simulink model "test"  (R2019a)
settings: Solver=VariableStepAuto  StartTime=0.0  StopTime=10.0  RelTol=1e-3
libraries: powerlib x9, re_lib x1, powerlib_meascontrol x1, ee_lib x1
settings Model: Creator=engma  LastModifiedBy=engma

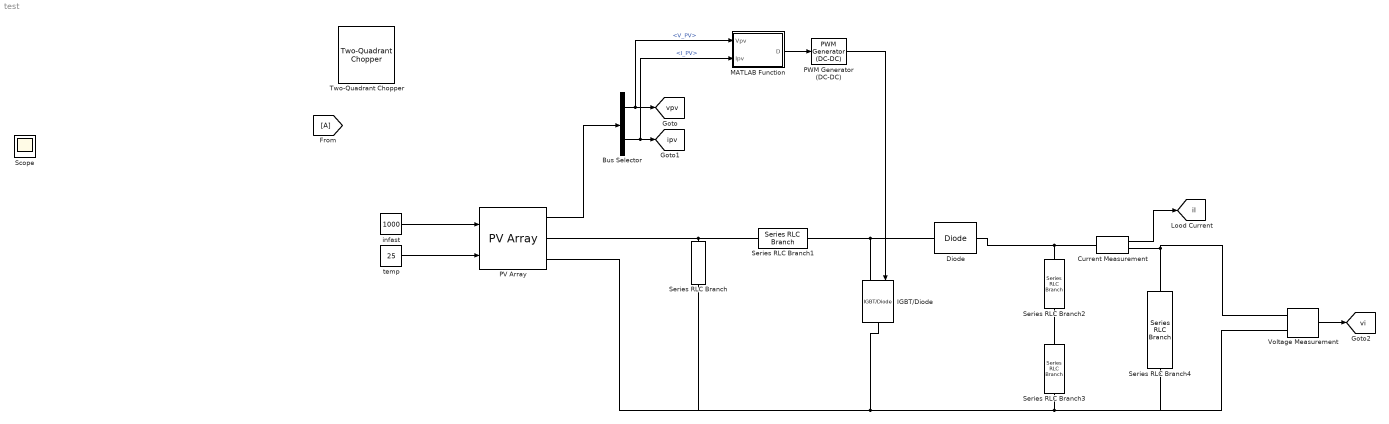
== system test ==
  Bus Selector : BusSelector  OutputSignals=V_PV,I_PV
  Current Measurement : powerlib/Measurements/Current Measurement  PhasorSimulation=off  OutputType=Complex  PSBequivalent=0
      settings: SourceProductName=Simscape Electrical
  Diode : powerlib/Power Electronics/Diode  Ron=0.001  Lon=0  Vf=0.8  IC=0  UseSnubber=0  Rs=500  Cs=250e-9  Measurements=off
      settings: SourceProductName=Simscape Electrical
  IGBT/Diode : powerlib/Power Electronics/IGBT//Diode  Ron=1e-3  Rs=1e5  Cs=inf  Measurements=off
      settings: SourceProductName=Simscape Electrical
  MATLAB Function : MATLAB Function  TreatAsAtomicUnit=on
  PV Array : re_lib/Solar/PV Array  Npar=64  Nser=5  PlotType=array @ 1000 W/m2 & specified temperatures  S_vec="[ 1000  500  100 ]"  Temp_C_vec="[ 45 25  ]"  ModuleName=1Soltech 1STH-215-P  PlotWhenSelected=off  Pm=213.15  Ncell=60  Voc=36.3  Isc=7.84  Vm=29  Im=7.35  beta_Voc_pc=-0.36099  alpha_Isc_pc=0.102  beta_Voc=-0.13104  alpha_Isc=0.007997  IL=7.8649  I0=2.9259e-10  nI=0.98117  Rsh=313.3991  Rs=0.39383  BAL=off  Tc=1e-6  Tfilter=5e-5
      settings: SourceProductName=Simscape Electrical
  PWM Generator (DC-DC) : powerlib_meascontrol/Pulse & Signal Generators/PWM Generator (DC-DC)  Fsw=5000  Ts=0
      settings: SourceProductName=Simscape Electrical
  Scope : Scope
  Series RLC Branch : powerlib/Elements/Series RLC Branch  LConnTagsString=__new0  RConnTagsString=__new0  BranchType=C  Resistance=1  Inductance=1e-3  SetiL0=off  InitialCurrent=0  Capacitance=100e-6  Setx0=off  InitialVoltage=0  Measurements=None
      settings: SourceProductName=Simscape Electrical
  Series RLC Branch1 : powerlib/Elements/Series RLC Branch  LConnTagsString=__new0  RConnTagsString=__new0  BranchType=L  Resistance=1  Inductance=1e-3  SetiL0=off  InitialCurrent=0  Capacitance=5e-3  Setx0=off  InitialVoltage=0  Measurements=None
      settings: SourceProductName=Simscape Electrical
  Series RLC Branch2 : powerlib/Elements/Series RLC Branch  LConnTagsString=__new0  RConnTagsString=__new0  BranchType=C  Resistance=1  Inductance=1e-3  SetiL0=off  InitialCurrent=0  Capacitance=12000e-6  Setx0=off  InitialVoltage=0  Measurements=None
      settings: SourceProductName=Simscape Electrical
  Series RLC Branch3 : powerlib/Elements/Series RLC Branch  LConnTagsString=__new0  RConnTagsString=__new0  BranchType=C  Resistance=1  Inductance=1e-3  SetiL0=off  InitialCurrent=0  Capacitance=12000e-6  Setx0=off  InitialVoltage=0  Measurements=None
      settings: SourceProductName=Simscape Electrical
  Series RLC Branch4 : powerlib/Elements/Series RLC Branch  LConnTagsString=__new0  RConnTagsString=__new0  BranchType=R  Resistance=10  Inductance=1e-3  SetiL0=off  InitialCurrent=0  Capacitance=12000e-6  Setx0=off  InitialVoltage=0  Measurements=None
      settings: SourceProductName=Simscape Electrical
  Two-Quadrant Chopper : ee_lib/Semiconductors & Converters/Converters/Two-Quadrant Chopper  device_type=2  Vf=0.8 V  Ron=0.001 Ohm  Rds=0.001 Ohm  Goff=1e-5 1/Ohm  Vth=6 V  Vgt=1 V  Vgt_off=-1 V  Ih=1 A  diode_param=2  diode_Vf=0.8 V  diode_Ron=0.001 Ohm  diode_Goff=1e-5 1/Ohm  diode_C=50 nF  diode_iRM=-235 A  diode_iF=300 A  diode_idot=-50 A/us  diode_trr_param=1  diode_trr_factor=3  diode_trr=15 us  diode_Qrr=1500 s*uA  snubber_type=0  Rs=0.1 Ohm  Cs=1e-7 F
      settings: SourceProductName=Simscape Electrical  SourceProductBaseCode=PS
  Voltage Measurement : powerlib/Measurements/Voltage Measurement  PhasorSimulation=off  OutputType=Complex  PSBequivalent=0
      settings: SourceProductName=Simscape Electrical
  infast : Constant  Value=1000
  temp : Constant  Value=25
  tag scope: il=global, ipv=global, vi=global, vpv=global
  wires:
  PV Array/1 -> Bus Selector/1
  infast/1 -> PV Array/1
  temp/1 -> PV Array/2
  Bus Selector/1 -> MATLAB Function/1(Vpv), [vpv]  "<V_PV>"
  Bus Selector/2 -> MATLAB Function/2(Ipv), [ipv]  "<I_PV>"
  Voltage Measurement/1 -> [vi]
  Current Measurement/1 -> [il]
  MATLAB Function/1(D) -> PWM Generator (DC-DC)/1
  PWM Generator (DC-DC)/1 -> IGBT/Diode/1
  connections:
  PV Array/RConn1 -- Series RLC Branch1/LConn1 -- Series RLC Branch/LConn1
  Series RLC Branch1/RConn1 -- Diode/LConn1 -- IGBT/Diode/LConn1
  Series RLC Branch3/RConn1 -- Series RLC Branch2/LConn1
  Series RLC Branch2/RConn1 -- Diode/RConn1 -- Current Measurement/LConn1
  IGBT/Diode/RConn1 -- Series RLC Branch/RConn1 -- PV Array/RConn2 -- Voltage Measurement/LConn2 -- Series RLC Branch4/LConn1 -- Series RLC Branch3/LConn1
  Series RLC Branch4/RConn1 -- Voltage Measurement/LConn1 -- Current Measurement/RConn1

== matlab function test/MATLAB Function ==
  data: Vpv input; D output; Ipv input
function D = PSO(Vpv,Ipv)

persistent u;
persistent dcurrent;
persistent pbest;
persistent p;            %power
persistent dc;           %duty cycle
persistent v;            %velocity
persistent counter;
persistent gbest;
% initialization :
if(isempty(counter))
    counter=0;          
    dcurrent=0.5;       %current duty cycle
    gbest=0.5;
    p=zeros(3,1);       %power
    v=zeros(3,1);       %voltage
    pbest=zeros(3,1);
    u=0;                
    dc=zeros(3,1);      %duty cycle
    %initial dc for each particle
    dc(1)=0.2;
    dc(2)=0.4;
    dc(3)=0.7;
    
end

% AT the first time , this if ignored (counter=0)
%Delay
if(counter>=1 && counter<300)
    D=dcurrent;
    counter=counter+1;
    return;                 %return control to the invoking function before it reaches the end of the function.
end
counter=0;                  %reset the counter 

%calculate the fittnes function (power) of each particle,
%then compare the current value of the function with previous one 
%if the current value is better than the previous ,update the value 
%Note: at the first time , this if ignored (u=0)
if(u>=1 && u<=3)
    if((Vpv*Ipv)>p(u))
        p(u)=Vpv*Ipv;
        pbest(u)=dcurrent;
    end
end


u=u+1;
% AT the first time , this if excuted  because it consist the condition...
% u==0(initial value of u)
if(u==5)
    u=1;
end

if(u==1)
    D=dc(u);
    dcurrent=D;
    counter=1;
    return;
elseif(u==2)
    D=dc(u);
    dcurrent=D;
    counter=1;
    return;
elseif(u==3)
    D=dc(u);
    dcurrent=D;
    counter=1;
    return;
elseif(u==4 )
    [m,i]=max(p);       %finds the indices of the maximum values of P (max power)and returns them in output vector i
    gbest=pbest(i);     % find the location(duty) of the particle which has max P 
    D=gbest;
    dcurrent=D;
    counter=1;
    %update velocity and duty cycle
    v(1)=updatevelocity(v(1),pbest(1),dc(1),gbest)
    v(2)=updatevelocity(v(2),pbest(2),dc(2),gbest)
    v(3)=updatevelocity(v(3),pbest(3),dc(3),gbest)
    
    %update duty cycle
    dc(1)=updateduty(dc(1),v(1))
    dc(2)=updateduty(dc(2),v(2))
    dc(3)=updateduty(dc(3),v(3))
    
    
    return;
    
else %if u==0 
   
    D=0.1;
    
end


end
function vfinal=updatevelocity(velocity,pobest,d,gwbest)
% PSO Parameters
w=0.4;
c1=1.2;         % Personal Learning Coefficient
c2=2;           % Global Learning Coefficient

vfinal = (w*velocity)+(c1*rand(1)*(pobest-d))+(c2*rand(1)*(gwbest-d));
end
function dfinal=updateduty(d,velocity)
dup=d+velocity;
if(dup>1)
    dfinal=1;
elseif(dup<0)
    dfinal=0;
else
    dfinal=dup;
end
end
